simulink model "rtwdemo_iec61508"  (Simulink 7.6)
settings: Solver=FixedStepDiscrete  SolverMode=SingleTasking  StartTime=0.0  StopTime=4  FixedStep=0.1  RelTol=1e-3  AbsTol=1e-6
InitFcn:
  | thr=40;
libraries: simulink x3, rtwdemowidgets x2
Description:
  | Using the IEC 61508 Modeling Standard Checks
  | This model demonstrates the Modeling Standard Checks for IEC 61508 in
  | Model Advisor. The IEC 61508 checks quickly identify issues with your model
  | that impede deployment in safety-critical applications or limit traceability.
settings Model: Creator=The MathWorks Inc.  CovMetricSettings=d  ExtModeTrigMode=oneshot  ExtModeArmWhenConnect=off  ExtModeAutoUpdateStatusClock=off
settings DataIOCC: LimitDataPoints=off  SaveOutput=off  SaveTime=off  SignalLoggingName=sigsOut
settings OptimizationCC: BlockReduction=off  InlineParams=on  InlineInvariantSignals=on  StateBitsets=on  DataBitsets=on  UseTempVars=on  ZeroExternalMemoryAtStartup=off  ZeroInternalMemoryAtStartup=off  EfficientFloat2IntCast=on  EfficientMapNaN2IntZero=off  OptimizeModelRefInitCode=on
settings DebuggingCC: AlgebraicLoopMsg=error  ArtificialAlgebraicLoopMsg=error  CheckExecutionContextPreStartOutputMsg=on  CheckExecutionContextRuntimeOutputMsg=on  BlockPriorityViolationMsg=error  SolverPrmCheckMsg=error  IntegerOverflowMsg=none  ParameterDowncastMsg=warning  ParameterOverflowMsg=warning  ParameterPrecisionLossMsg=none  UnnecessaryDatatypeConvMsg=warning  SignalLabelMismatchMsg=error  UnconnectedInputMsg=error  UnconnectedOutputMsg=error  UnconnectedLineMsg=error  UnknownTsInhSupMsg=error  StrictBusMsg=ErrorOnBusTreatedAsVector
settings HardwareCC: ProdIntDivRoundTo=Zero  ProdEndianess=LittleEndian  ProdHWDeviceType=Generic->32-bit Embedded Processor  TargetHWDeviceType=Generic->32-bit Embedded Processor
settings SFSimCC: SimParseCustomCode=off
settings RTWCC: SystemTargetFile=ert.tlc  GenCodeOnly=on  TemplateMakefile=ert_default_tmf  Description=Real-Time Workshop Embedded Coder (no auto configuration)  GenerateReport=on  RTWVerbose=off  ProcessScript=ert_make_rtw_hook  IncludeHyperlinkInReport=on  LaunchReport=on  GenerateTraceInfo=on  GenerateTraceReport=on  GenerateTraceReportSl=on  GenerateTraceReportSf=on  GenerateTraceReportEml=on
settings CodeAppCC: ForceParamTrailComments=on  IgnoreCustomStorageClasses=off  IncHierarchyInIds=on  SimulinkDataObjDesc=on  IncDataTypeInIds=on  CustomSymbolStrGlobalVar=rt$N$M  CustomSymbolStrType=$N$M  CustomSymbolStrFcn=$N$M$F  CustomSymbolStrMacro=$N$M  InsertBlockDesc=on  ReqsInCode=on
settings ERTTargetCC: MultiwordLength=2048  GenerateSampleERTMain=on  IncludeMdlTerminateFcn=off  SupportNonFinite=off  SupportComplex=off  InlinedParameterPlacement=NonHierarchical  ERTCustomFileTemplate=example_file_process.tlc  ConvertIfToSwitch=off

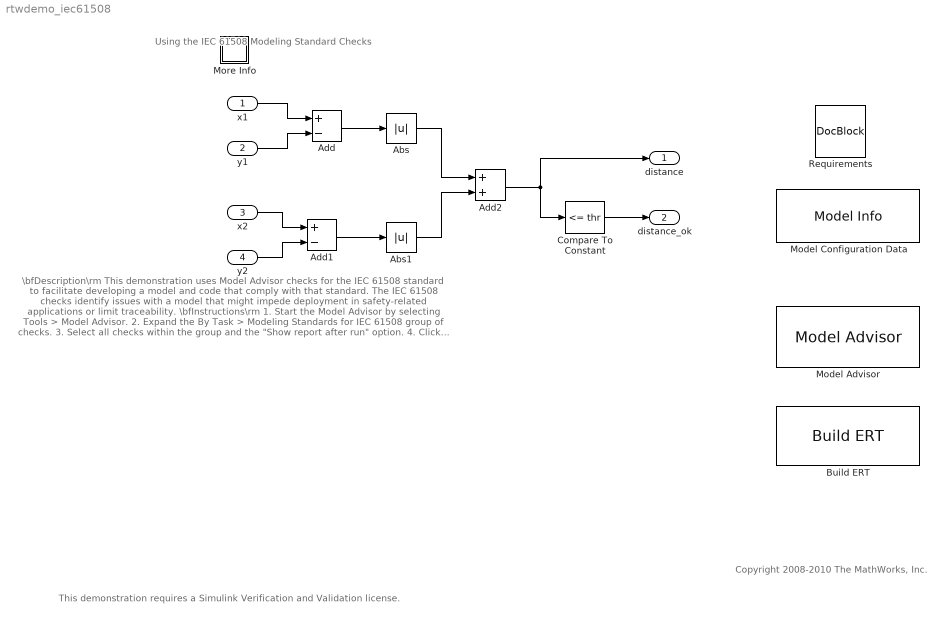
== system rtwdemo_iec61508 ==
  note: \bfDescription\rm
      | This demonstration uses Model Advisor checks for the IEC 61508
      | standard to facilitate developing a model and code that comply with that
      | standard. The IEC 61508 checks identify issues with a model that might
      |  impede deployment in safety-related applications or limit traceability.
      |
      | \bfInstructions\rm
      | 1. Start the Model Advisor by selecting Tools > Model Advisor.
      | 2. Expand the By Task > Modeling Standards for IEC 61508 group of checks.
      | 3. Select all checks within the group and the "Show report after run" option.
      | 4. Click the Run Selected Checks button.
      | 5. Inspect the check results and the generated Model Advisor report.
      | 6. Fix reported issues.
      | 7. Rerun the checks.
      |
      | Double-click the Launch Model Advisor button to automate step 1.
      | Double-click the Generate Code Using Real-Time Workshop Embedded Coder
      | button to generate source code and open the code generation HTML report.
  note: Copyright 2008-2010 The MathWorks, Inc.
  note: Using the IEC 61508 Modeling Standard Checks
  note: This demonstration requires a Simulink Verification and Validation license.
  x1 : Inport  OutDataTypeStr=uint16  Interpolate=off
  y1 : Inport  Port=2  OutDataTypeStr=uint16  Interpolate=off
  x2 : Inport  Port=3  OutDataTypeStr=int16  Interpolate=off
  y2 : Inport  Port=4  OutDataTypeStr=int16  Interpolate=off
  Abs : Abs
  Abs1 : Abs  SaturateOnIntegerOverflow=on
  Add : Sum  Inputs=+-
  Add1 : Sum  Inputs=+-
  Add2 : Sum  OutDataTypeStr=int16
  Build ERT : rtwdemowidgets/Build ERT  SystemSampleTime=-1  attrib_overrides={'BlockReduction' 'LifeSpan' 'EnforceIntegerDowncast' 'NoFixptDivByZeroProtection'}
  Compare To Constant : simulink/Logic and Bit Operations/Compare To Constant  SystemSampleTime=-1  relop=<=  const=thr  LogicOutDataTypeMode=boolean  ZeroCross=off
  Model Advisor : rtwdemowidgets/Model Advisor  SystemSampleTime=-1  attrib_overrides={}
  Model Configuration Data : simulink/Model-Wide Utilities/Model Info  SystemSampleTime=-1  InitialBlockCM=none  BlockCM=none  Frame=on  DisplayStringWithTags=|  HorizontalTextAlignment=Left  LeftAlignmentValue=0.02  SourceBlockDiagram=rtwdemo_iec61508  TagMaxNumber=20
      | Model version: %<ModelVersion>
      | Author: %<LastModifiedBy>
      | Date: %<LastModificationDate>
  More Info : Subsystem
      settings: OpenFcn=showdemo('rtwdemo_iec61508_script')
      mask Display: disp('?')
  Requirements : simulink/Model-Wide Utilities/DocBlock  SystemSampleTime=-1  ECoderFlag=y  DocumentType=Text
      content=|
      | Check if the 1-norm distance between the points (x1, x2) and (y1, y2) is less or equal than a given threshold thr.
      |
      | For two points (x1, x2) and (y1, y2) the 1-norm distance is given as |x1-y1| + |x2-y2|
  distance : Outport
  distance_ok : Outport  Port=2
  wires:
  x1/1 -> Add/1
  y1/1 -> Add/2
  x2/1 -> Add1/1
  y2/1 -> Add1/2
  Add/1 -> Abs/1
  Add1/1 -> Abs1/1
  Abs1/1 -> Add2/2
  Add2/1 -> Compare To Constant/1, distance/1
  Compare To Constant/1 -> distance_ok/1
  Abs/1 -> Add2/1

== system rtwdemo_iec61508/More Info ==
